simulink model "incidence_angle_test"  (R2020b)
settings: Solver=VariableStepAuto  StartTime=0.0  StopTime=10.0  RelTol=1e-3
libraries: aerolibasang x1
settings Model: Creator=natha  LastModifiedBy=natha

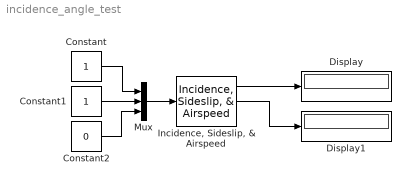
== system incidence_angle_test ==
  Constant : Constant
  Constant1 : Constant
  Constant2 : Constant  Value=0
  Display : Display
  Display1 : Display
  "Incidence, Sideslip, & Airspeed" : aerolibasang/Incidence, Sideslip, & Airspeed
  Mux : Mux  Inputs=3
  wires:
  "Incidence, Sideslip, & Airspeed"/1 -> Display/1
  Mux/1 -> "Incidence, Sideslip, & Airspeed"/1
  Constant/1 -> Mux/1
  Constant2/1 -> Mux/3
  Constant1/1 -> Mux/2
  "Incidence, Sideslip, & Airspeed"/2 -> Display1/1
